simulink model "untitled"  (Simulink 7.5)
settings: Solver=ode45  StartTime=0.0  StopTime=100  RelTol=1e-3
settings Model: Creator=jlu  LastModifiedBy=jlu

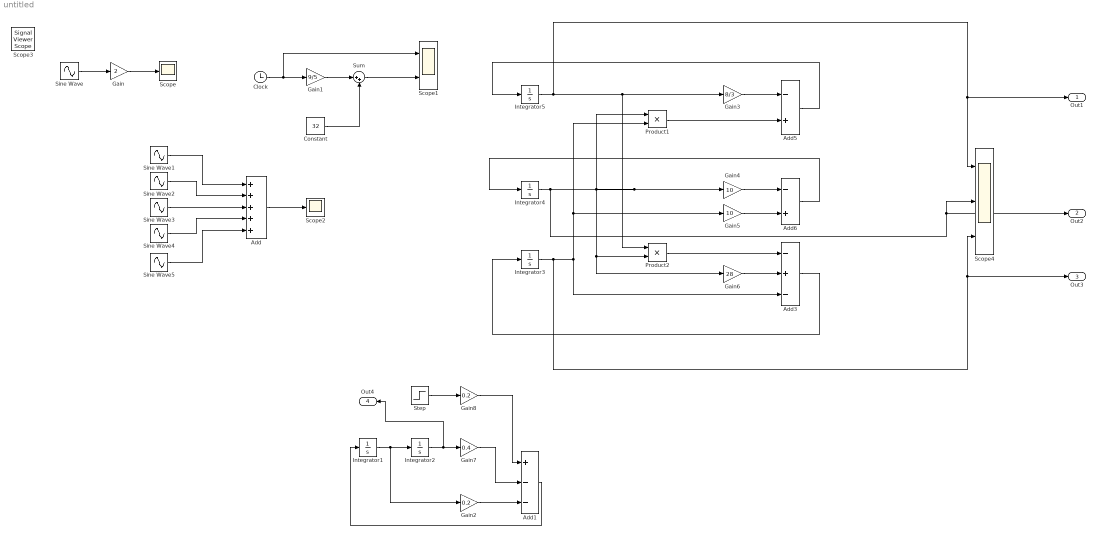
== system untitled ==
  Add : Sum  Inputs=+++++  OutDataType=fixdt(1, 16)  OutScaling=2^-10
  Add1 : Sum  Inputs=+--  OutDataType=fixdt(1, 16)  OutScaling=2^-10
  Add3 : Sum  Inputs=-+-  OutDataType=fixdt(1, 16)  OutScaling=2^-10
  Add5 : Sum  Inputs=-+  OutDataType=fixdt(1, 16)  OutScaling=2^-10
  Add6 : Sum  Inputs=-+  OutDataType=fixdt(1, 16)  OutScaling=2^-10
  Clock : Clock
      settings: Decimation=10
  Constant : Constant  Value=32  OutDataType=fixdt(1, 16)  OutScaling=2^0
  Gain : Gain  Gain=2  ParameterDataType=fixdt(1, 16)  ParameterScaling=2^0  OutDataType=fixdt(1, 16)  OutScaling=2^0
  Gain1 : Gain  Gain=9/5  ParameterDataType=fixdt(1, 16)  ParameterScaling=2^0  OutDataType=fixdt(1, 16)  OutScaling=2^0
  Gain2 : Gain  Gain=0.2  ParameterDataType=fixdt(1, 16)  ParameterScaling=2^0  OutDataType=fixdt(1, 16)  OutScaling=2^0
  Gain3 : Gain  Gain=8/3  ParameterDataType=fixdt(1, 16)  ParameterScaling=2^0  OutDataType=fixdt(1, 16)  OutScaling=2^0
  Gain4 : Gain  Gain=10  ParameterDataType=fixdt(1, 16)  ParameterScaling=2^0  OutDataType=fixdt(1, 16)  OutScaling=2^0
  Gain5 : Gain  Gain=10  ParameterDataType=fixdt(1, 16)  ParameterScaling=2^0  OutDataType=fixdt(1, 16)  OutScaling=2^0
  Gain6 : Gain  Gain=28  ParameterDataType=fixdt(1, 16)  ParameterScaling=2^0  OutDataType=fixdt(1, 16)  OutScaling=2^0
  Gain7 : Gain  Gain=0.4  ParameterDataType=fixdt(1, 16)  ParameterScaling=2^0  OutDataType=fixdt(1, 16)  OutScaling=2^0
  Gain8 : Gain  Gain=0.2  ParameterDataType=fixdt(1, 16)  ParameterScaling=2^0  OutDataType=fixdt(1, 16)  OutScaling=2^0
  Integrator{1..5} (5 alike) : Integrator  InitialCondition=1e-10
  Product1 : Product  OutDataType=fixdt(1, 16)  OutScaling=2^0  RndMeth=Zero
  Product2 : Product  OutDataType=fixdt(1, 16)  OutScaling=2^0  RndMeth=Zero
  Scope : Scope
  Scope1 : Scope  NumInputPorts=2
      settings: YMin=-5~-5  YMax=5~5
  Scope2 : Scope
      settings: TimeRange=4.494933636411957e-008  YMin=1.347364300399846  YMax=1.407046227116923  SaveName=ScopeData2
  Scope4 : Scope  NumInputPorts=3
      settings: TimeRange=4.494933636411957e-008  YMin=1.34736~-5~-5  YMax=1.40705~5~5  SaveName=ScopeData3
  Sine Wave : Sin  Amplitude=1  Bias=0  Frequency=1  Phase=0  Samples=10  SampleTime=0  Offset=0
  Sine Wave1 : Sin  Amplitude=1  Bias=0  Frequency=2*pi  Phase=0  Samples=10  SampleTime=0  Offset=0
  Sine Wave2 : Sin  Amplitude=1/3  Bias=0  Frequency=2*pi*3  Phase=0  Samples=10  SampleTime=0  Offset=0
  Sine Wave3 : Sin  Amplitude=1/5  Bias=0  Frequency=2*pi*5  Phase=0  Samples=10  SampleTime=0  Offset=0
  Sine Wave4 : Sin  Amplitude=1/7  Bias=0  Frequency=2*pi*7  Phase=0  Samples=10  SampleTime=0  Offset=0
  Sine Wave5 : Sin  Amplitude=9/1  Bias=0  Frequency=2*pi*9  Phase=0  Samples=10  SampleTime=0  Offset=0
  Step : Step  SampleTime=0
  Sum : Sum  Inputs=|++  OutDataType=fixdt(1, 16)  OutScaling=2^0
  Out1 : Outport  OutDataType=fixdt(1, 16)  OutScaling=2^0
  Out2 : Outport  Port=2  OutDataType=fixdt(1, 16)  OutScaling=2^0
  Out3 : Outport  Port=3  OutDataType=fixdt(1, 16)  OutScaling=2^0
  Out4 : Outport  Port=4  OutDataType=fixdt(1, 16)  OutScaling=2^0
  Scope3 : SignalViewerScope  IOType=viewer  RefreshTime=0.035000
  wires:
  Sine Wave/1 -> Gain/1
  Gain/1 -> Scope/1
  Gain1/1 -> Sum/1
  Constant/1 -> Sum/2
  Sum/1 -> Scope1/2
  Clock/1 -> Gain1/1, Scope1/1
  Sine Wave1/1 -> Add/1
  Sine Wave2/1 -> Add/2
  Sine Wave3/1 -> Add/3
  Sine Wave4/1 -> Add/4
  Sine Wave5/1 -> Add/5
  Add/1 -> Scope2/1
  Integrator3/1 -> Add3/3, Product1/2, Gain5/1, Scope4/3, Out3/1
  Integrator4/1 -> Product1/1, Gain4/1, Product2/2, Gain6/1, Scope4/2, Out2/1
  Integrator5/1 -> Gain3/1, Product2/1, Scope4/1, Out1/1
  Add5/1 -> Integrator5/1
  Add6/1 -> Integrator4/1
  Gain3/1 -> Add5/1
  Product1/1 -> Add5/2
  Gain4/1 -> Add6/1
  Gain5/1 -> Add6/2
  Product2/1 -> Add3/1
  Gain6/1 -> Add3/2
  Add3/1 -> Integrator3/1
  Integrator1/1 -> Integrator2/1, Gain2/1
  Gain2/1 -> Add1/3
  Integrator2/1 -> Gain7/1, Out4/1
  Gain7/1 -> Add1/2
  Gain8/1 -> Add1/1
  Add1/1 -> Integrator1/1
  Step/1 -> Gain8/1
